simulink model "BLSMC"  (R2025b)
settings: Solver=ode3  StartTime=0.0  StopTime=1.5  FixedStep=1e-5  RelTol=1e-3  EnableMultiTasking=on
values from neighbouring files (symbols this model uses):
  beta = 2e3    (= 2000)    [plotting.m]    (also in robusnost_grafici.m)
  C = 470*10^-6    (= 0.00047)    [plotting.m]    (also in robusnost_grafici.m)
  k0 = 2*200    (= 400)    [plotting.m]    (also in robusnost_grafici.m)
  k1 = 1    [plotting.m]    (also in robusnost_grafici.m)
  ki = 200^2    (= 40000)    [plotting.m]    (also in robusnost_grafici.m)
  L = 15.91*10^-3    (= 0.01591)    [plotting.m]    (also in robusnost_grafici.m = 0.012728)
  poremecaj = 0.8    [plotting.m]    (also in robusnost_grafici.m)
  R = 52    [plotting.m]    (also in robusnost_grafici.m)
  sel = 3    [plotting.m]    (also in robusnost_grafici.m)
  sig2 = (0.02*x2e)^2    (= 0.2025)    [plotting.m]    (also in robusnost_grafici.m = 0)
  wp = 150    [plotting.m]    (also in robusnost_grafici.m)
  x2e = Vc    (= -22.5)    [plotting.m]    (also in robusnost_grafici.m)
settings Model: Creator=Stevica  LastModifiedBy=User
settings SolverCC: AlgebraicLoopSolver=TrustRegion
settings DataIOCC: LimitDataPoints=on  SaveFormat=Array
settings OptimizationCC: LifeSpan=inf
settings DebuggingCC: UnderspecifiedInitializationDetection=Classic  MergeDetectMultiDrivingBlocksExec=none  SolverPrmCheckMsg=warning  UnconnectedInputMsg=warning  UnconnectedOutputMsg=warning  UnconnectedLineMsg=warning  SFUnexpectedBacktrackingDiag=warning  SFNoUnconditionalDefaultTransitionDiag=warning  SFExecutionAtInitializationDiag=none  ArithmeticOperatorsInVariantConditions=warning
settings HardwareCC: ProdBitPerPointer=32.0  ProdBitPerSizeT=32.0  ProdBitPerPtrDiffT=32.0  ProdLargestAtomicFloat=None  ProdIntDivRoundTo=Undefined  ProdEndianess=Unspecified  ProdWordSize=32.0  ProdHWDeviceType=32-bit Generic
settings ModelReferenceCC: PropagateSignalLabelsOutOfModel=off
settings SFSimCC: SimUseLocalCustomCode=off  CustomCodeUndefinedFunction=UseInterfaceOnly
settings RTWCC: RTWUseLocalCustomCode=off  GPUComputeCapability=3.5
settings CodeAppCC: StateflowObjectComments=on
settings GRTTargetCC: TargetLangStandard=C89/C90 (ANSI)
settings ConfigComp: CovMetricSettings=dw  CovSaveCumulativeToWorkspaceVar=on  CovSaveSingleToWorkspaceVar=on  CovExternalEMLEnable=off

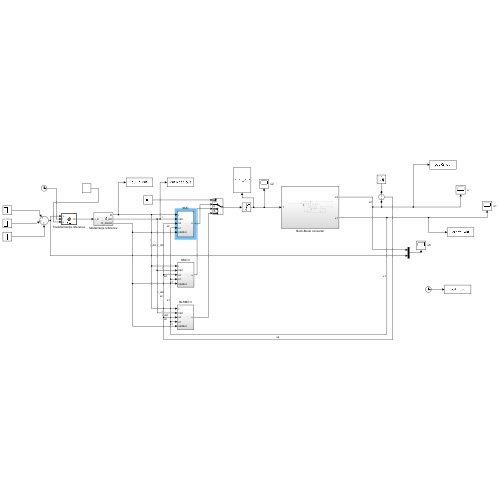
[thumbnail: Simulink's stored preview of the top-level diagram]
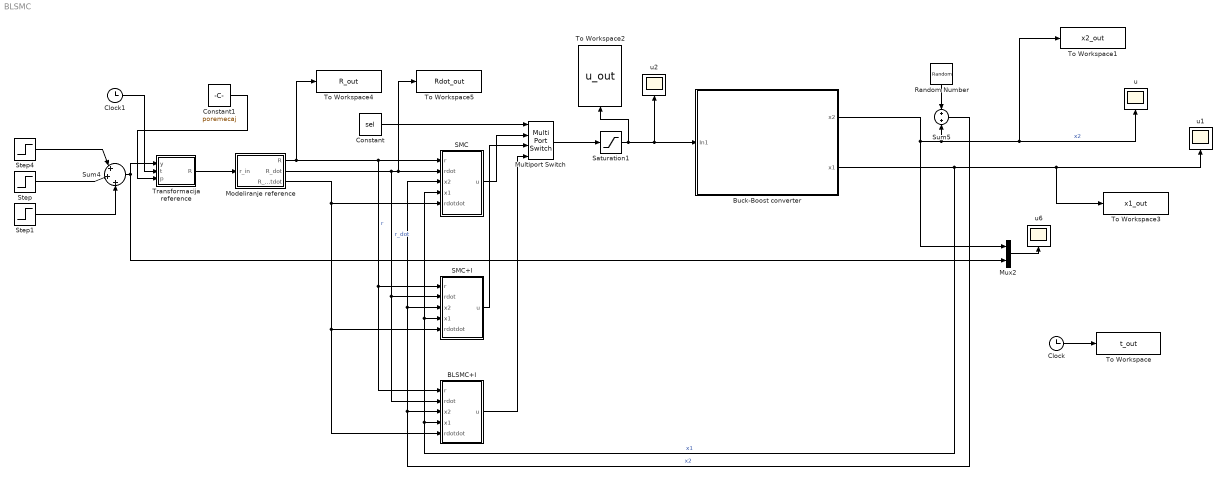
== system BLSMC ==
  BLSMC+I : Subsystem
      settings: PortSchema="{\"entries\":[{\"content\":{\"sides\":[{\"content\":{\"connectorIds\":[\"Out1\"]},\"type\":\"ConnectorPlacement.EquallySpacedRectSide\",\"uuid\":\"fc4d1246-7468-4525-a5ed-aeaa813f79b9\"},{\"content\":{\"connectorIds\":[\"In1\",\"In2\",\"In3\",\"In4\",\"In5\"],\"side\":\"RIGHT\"},\"type\":\"ConnectorPlacement.EquallySpacedRectSide\",\"uuid\":\"043d6a8f-e326-4119-9507-3ed5a55de0f4\"},{\"content\":{\"side\":\"TOP\"},\"type\":\"ConnectorPlacement.EquallySpacedRectSide\",\"uuid\":\"52d26304-56e6-4b52-8faf-a8e357024c95\"}]},\"type\":\"ConnectorPlacement.EquallySpacedConnector\",\"uuid\":\"d1c4fd68-439c-47cf-b9bf-33c74b646101\"}],\"packageUris\":[\"http://schema.mathworks.com/mf0/Connector/R2020b\"],\"version\":\"1.0\"}"
  Buck-Boost converter : Subsystem
  Clock : Clock
  Clock1 : Clock
  Constant : Constant  Value=sel
  Constant1 : Constant  Value=poremecaj
  Modeliranje reference : Subsystem
  Multiport Switch : MultiPortSwitch  SaturateOnIntegerOverflow=off  InputSameDT=off
  Mux2 : Mux  Inputs=2
  Random Number : RandomNumber  Variance=sig2  SampleTime=1e-5
  SMC : Subsystem
      settings: PortSchema="{\"entries\":[{\"content\":{\"sides\":[{\"content\":{\"connectorIds\":[\"Out1\"]},\"type\":\"ConnectorPlacement.EquallySpacedRectSide\",\"uuid\":\"fc4d1246-7468-4525-a5ed-aeaa813f79b9\"},{\"content\":{\"connectorIds\":[\"In1\",\"In2\",\"In3\",\"In4\",\"In5\"],\"side\":\"RIGHT\"},\"type\":\"ConnectorPlacement.EquallySpacedRectSide\",\"uuid\":\"043d6a8f-e326-4119-9507-3ed5a55de0f4\"},{\"content\":{\"side\":\"TOP\"},\"type\":\"ConnectorPlacement.EquallySpacedRectSide\",\"uuid\":\"52d26304-56e6-4b52-8faf-a8e357024c95\"}]},\"type\":\"ConnectorPlacement.EquallySpacedConnector\",\"uuid\":\"d1c4fd68-439c-47cf-b9bf-33c74b646101\"}],\"packageUris\":[\"http://schema.mathworks.com/mf0/Connector/R2020b\"],\"version\":\"1.0\"}"
  SMC+I : Subsystem
      settings: PortSchema="{\"entries\":[{\"content\":{\"sides\":[{\"content\":{\"connectorIds\":[\"Out1\"]},\"type\":\"ConnectorPlacement.EquallySpacedRectSide\",\"uuid\":\"fc4d1246-7468-4525-a5ed-aeaa813f79b9\"},{\"content\":{\"connectorIds\":[\"In1\",\"In2\",\"In3\",\"In4\",\"In5\"],\"side\":\"RIGHT\"},\"type\":\"ConnectorPlacement.EquallySpacedRectSide\",\"uuid\":\"043d6a8f-e326-4119-9507-3ed5a55de0f4\"},{\"content\":{\"side\":\"TOP\"},\"type\":\"ConnectorPlacement.EquallySpacedRectSide\",\"uuid\":\"52d26304-56e6-4b52-8faf-a8e357024c95\"}]},\"type\":\"ConnectorPlacement.EquallySpacedConnector\",\"uuid\":\"d1c4fd68-439c-47cf-b9bf-33c74b646101\"}],\"packageUris\":[\"http://schema.mathworks.com/mf0/Connector/R2020b\"],\"version\":\"1.0\"}"
  Saturation1 : Saturate  UpperLimit=1  LowerLimit=0
  Step : Step  Time=0.5  After=5  SampleTime=0
  Step1 : Step  After=-5  SampleTime=0
  Step4 : Step  Time=0  After=x2e  SampleTime=0
  Sum4 : Sum  Inputs=|+|+|+
  Sum5 : Sum
  To Workspace : ToWorkspace  VariableName=t_out  SampleTime=-1
  To Workspace1 : ToWorkspace  VariableName=x2_out  SampleTime=-1
  To Workspace2 : ToWorkspace  VariableName=u_out  SampleTime=-1
  To Workspace3 : ToWorkspace  VariableName=x1_out  SampleTime=-1
  To Workspace4 : ToWorkspace  VariableName=R_out  SampleTime=-1
  To Workspace5 : ToWorkspace  VariableName=Rdot_out  SampleTime=-1
  Transformacija reference : MATLAB Function  TreatAsAtomicUnit=on
  u{,1..2,6} (4 alike) : Scope
      u settings: ActiveDisplayYMinimum=-24.287940428418956  ActiveDisplayYMaximum=-16.345568269350679
      u1 settings: ActiveDisplayYMinimum=-0.56796240385681784  ActiveDisplayYMaximum=46.459814294123959
      u2 settings: ActiveDisplayYMinimum=0.31863871310778108  ActiveDisplayYMaximum=0.92761461889170183  DataLoggingVariableName=ScopeData3
      u6 settings: ActiveDisplayYMinimum=-24.906803320525466  ActiveDisplayYMaximum=-19.322890473907805  DataLoggingVariableName=ScopeData8
  wires:
  Buck-Boost converter/2(x1) -> To Workspace3/1, u1/1, BLSMC+I/4(x1), SMC/4(x1), SMC+I/4(x1)  "x1"
  Saturation1/1 -> Buck-Boost converter/1(In1), u2/1, To Workspace2/1
  Sum4/1 -> Mux2/2, Transformacija reference/1(y)
  Step/1 -> Sum4/2
  Step1/1 -> Sum4/3
  Sum5/1 -> BLSMC+I/3(x2), SMC/3(x2), SMC+I/3(x2)  "x2"
  Mux2/1 -> u6/1
  Step4/1 -> Sum4/1
  SMC/1(u) -> Multiport Switch/2
  Multiport Switch/1 -> Saturation1/1
  Modeliranje reference/1(R) -> To Workspace4/1, BLSMC+I/1(r), SMC+I/1(r), SMC/1(r)  "r"
  Modeliranje reference/2(R_dot) -> To Workspace5/1, SMC/2(rdot), BLSMC+I/2(rdot), SMC+I/2(rdot)  "r_dot"
  SMC+I/1(u) -> Multiport Switch/3
  BLSMC+I/1(u) -> Multiport Switch/4
  Constant/1 -> Multiport Switch/1
  Modeliranje reference/3(R_dotdot) -> SMC+I/5(rdotdot), BLSMC+I/5(rdotdot), SMC/5(rdotdot)
  Random Number/1 -> Sum5/1
  Buck-Boost converter/1(x2) -> Mux2/1, To Workspace1/1, u/1, Sum5/2  "x2"
  Clock/1 -> To Workspace/1
  Transformacija reference/1(R) -> Modeliranje reference/1(r_in)
  Clock1/1 -> Transformacija reference/2(t)
  Constant1/1 -> Transformacija reference/3(p)

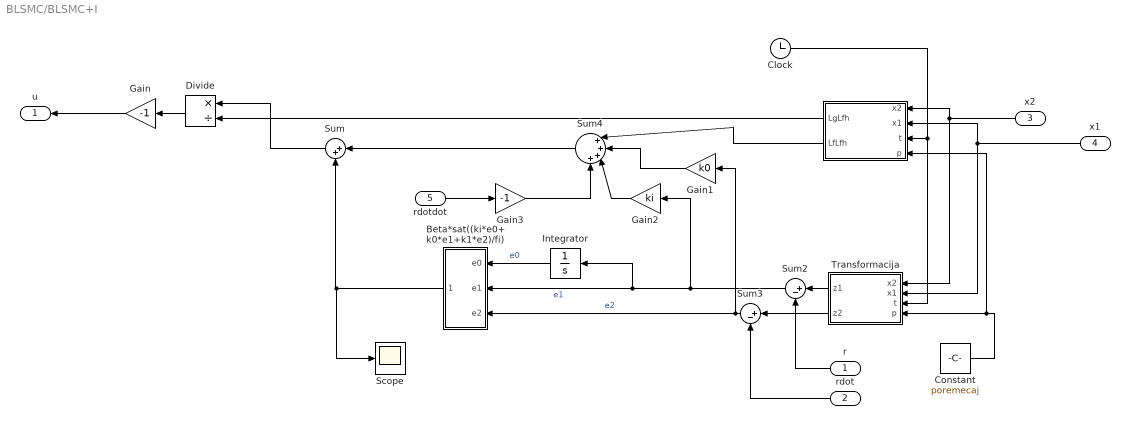
== system BLSMC/BLSMC+I ==
  r : Inport
  rdot : Inport  Port=2
  x2 : Inport  Port=3
  x1 : Inport  Port=4
  rdotdot : Inport  Port=5
  " " : MATLAB Function  TreatAsAtomicUnit=on
  Beta*sat((ki*e0+ k0*e1+k1*e2)/fi) : Subsystem
  Clock : Clock
  Constant : Constant  Value=poremecaj
  Divide : Product  Inputs=*/
  Gain : Gain  Gain=-1
  Gain1 : Gain  Gain=k0
  Gain2 : Gain  Gain=ki
  Gain3 : Gain  Gain=-1
  Integrator : Integrator
  Scope : Scope
      settings: ActiveDisplayYMinimum=-2170.4046249704252  ActiveDisplayYMaximum=-1714.2392861068972  DataLoggingVariableName=ScopeData4
  Sum : Sum  Inputs=|++
  Sum2 : Sum  Inputs=|+-
  Sum3 : Sum  Inputs=|+-
  Sum4 : Sum  Inputs=|++++
  Transformacija : MATLAB Function  TreatAsAtomicUnit=on
  u : Outport
  wires:
  Transformacija/1(z1) -> Sum2/1
  x2/1 -> Transformacija/1(x2), " "/1(x2)
  x1/1 -> Transformacija/2(x1), " "/2(x1)
  Transformacija/2(z2) -> Sum3/1
  Sum3/1 -> Gain1/1, Beta*sat((ki*e0+ k0*e1+k1*e2)/fi)/3(e2)  "e2"
  r/1 -> Sum2/2
  rdot/1 -> Sum3/2
  " "/2(LfLfh) -> Sum4/1
  Gain1/1 -> Sum4/2
  Sum4/1 -> Sum/1
  Sum2/1 -> Gain2/1, Integrator/1, Beta*sat((ki*e0+ k0*e1+k1*e2)/fi)/2(e1)  "e1"
  Beta*sat((ki*e0+ k0*e1+k1*e2)/fi)/1(Out1) -> Scope/1, Sum/2
  Sum/1 -> Divide/1
  " "/1(LgLfh) -> Divide/2
  Divide/1 -> Gain/1
  Gain/1 -> u/1
  Integrator/1 -> Beta*sat((ki*e0+ k0*e1+k1*e2)/fi)/1(e0)  "e0"
  Gain2/1 -> Sum4/3
  rdotdot/1 -> Gain3/1
  Gain3/1 -> Sum4/4
  Clock/1 -> Transformacija/3(t), " "/3(t)
  Constant/1 -> " "/4(p), Transformacija/4(p)

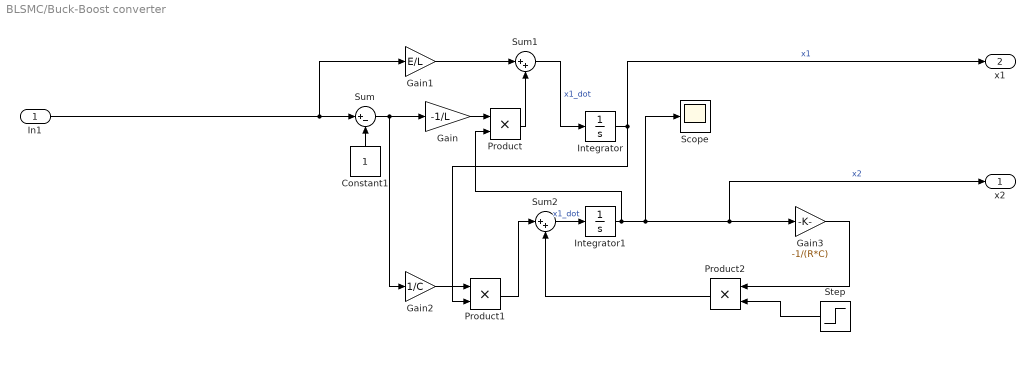
== system BLSMC/Buck-Boost converter ==
  In1 : Inport
  Constant1 : Constant
  Gain : Gain  Gain=-1/L
  Gain1 : Gain  Gain=E/L
  Gain2 : Gain  Gain=1/C
  Gain3 : Gain  Gain=-1/(R*C)
  Integrator : Integrator
  Integrator1 : Integrator
  Product : Product
  Product1 : Product
  Product2 : Product
  Scope : Scope
      settings: ActiveDisplayYMinimum=-25.046281735862888  ActiveDisplayYMaximum=-15.447926718255747  DataLoggingVariableName=ScopeData8
  Step : Step  Time=1.3  Before=1  After=1/poremecaj  SampleTime=0
  Sum : Sum  Inputs=|+-
  Sum1 : Sum  Inputs=|++
  Sum2 : Sum  Inputs=|++
  x2 : Outport
  x1 : Outport  Port=2
  wires:
  Gain/1 -> Product/1
  In1/1 -> Gain1/1, Sum/1
  Sum1/1 -> Integrator/1  "x1_dot"
  Gain1/1 -> Sum1/1
  Sum/1 -> Gain2/1, Gain/1
  Constant1/1 -> Sum/2
  Gain2/1 -> Product1/1
  Product/1 -> Sum1/2
  Integrator1/1 -> x2/1, Gain3/1, Scope/1, Product/2  "x2"
  Product1/1 -> Sum2/1
  Integrator/1 -> x1/1, Product1/2  "x1"
  Sum2/1 -> Integrator1/1  "x1_dot"
  Gain3/1 -> Product2/1
  Product2/1 -> Sum2/2
  Step/1 -> Product2/2

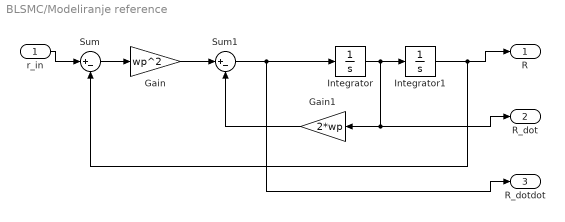
== system BLSMC/Modeliranje reference ==
  r_in : Inport
  Gain : Gain  Gain=wp^2
  Gain1 : Gain  Gain=2*wp
  Integrator : Integrator
  Integrator1 : Integrator
  Sum : Sum  Inputs=|+-
  Sum1 : Sum  Inputs=|+-
  R : Outport
  R_dot : Outport  Port=2
  R_dotdot : Outport  Port=3
  wires:
  r_in/1 -> Sum/1
  Sum/1 -> Gain/1
  Gain/1 -> Sum1/1
  Integrator/1 -> R_dot/1, Gain1/1, Integrator1/1
  Integrator1/1 -> Sum/2, R/1
  Gain1/1 -> Sum1/2
  Sum1/1 -> R_dotdot/1, Integrator/1

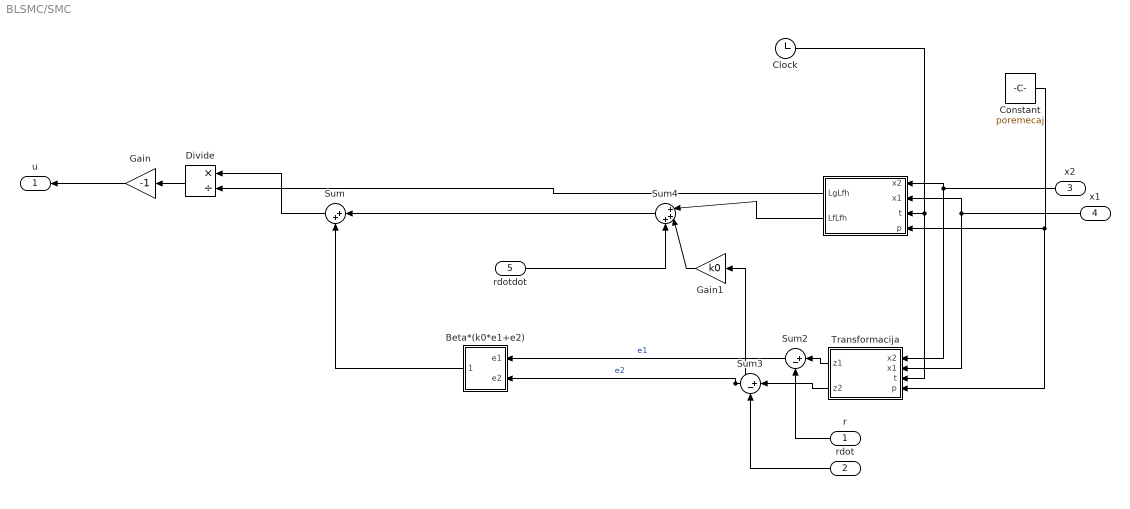
== system BLSMC/SMC ==
  r : Inport
  rdot : Inport  Port=2
  x2 : Inport  Port=3
  x1 : Inport  Port=4
  rdotdot : Inport  Port=5
  " " : MATLAB Function  TreatAsAtomicUnit=on
  Beta*(k0*e1+e2) : Subsystem
  Clock : Clock
  Constant : Constant  Value=poremecaj
  Divide : Product  Inputs=*/
  Gain : Gain  Gain=-1
  Gain1 : Gain  Gain=k0
  Sum : Sum  Inputs=|++
  Sum2 : Sum  Inputs=|+-
  Sum3 : Sum  Inputs=|+-
  Sum4 : Sum  Inputs=|+++
  Transformacija : MATLAB Function  TreatAsAtomicUnit=on
  u : Outport
  wires:
  Transformacija/1(z1) -> Sum2/1
  x2/1 -> Transformacija/1(x2), " "/1(x2)
  x1/1 -> " "/2(x1), Transformacija/2(x1)
  Transformacija/2(z2) -> Sum3/1
  Sum3/1 -> Beta*(k0*e1+e2)/2(e2), Gain1/1  "e2"
  r/1 -> Sum2/2
  rdot/1 -> Sum3/2
  " "/2(LfLfh) -> Sum4/1
  Gain1/1 -> Sum4/2
  Sum4/1 -> Sum/1
  Sum2/1 -> Beta*(k0*e1+e2)/1(e1)  "e1"
  Beta*(k0*e1+e2)/1(Out1) -> Sum/2
  Sum/1 -> Divide/1
  " "/1(LgLfh) -> Divide/2
  Divide/1 -> Gain/1
  Gain/1 -> u/1
  rdotdot/1 -> Sum4/3
  Clock/1 -> Transformacija/3(t), " "/3(t)
  Constant/1 -> Transformacija/4(p), " "/4(p)

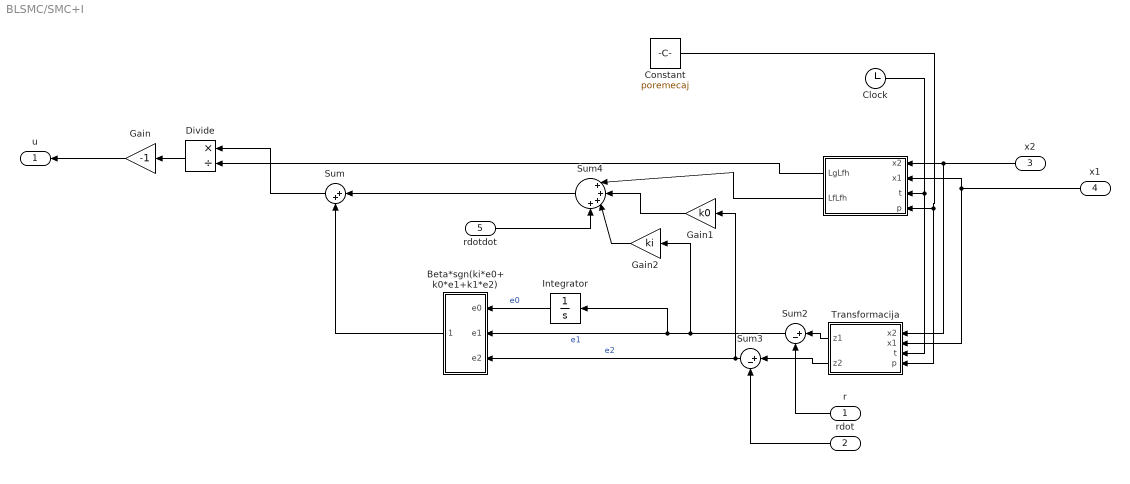
== system BLSMC/SMC+I ==
  r : Inport
  rdot : Inport  Port=2
  x2 : Inport  Port=3
  x1 : Inport  Port=4
  rdotdot : Inport  Port=5
  " " : MATLAB Function  TreatAsAtomicUnit=on
  Beta*sgn(ki*e0+ k0*e1+k1*e2) : Subsystem
  Clock : Clock
  Constant : Constant  Value=poremecaj
  Divide : Product  Inputs=*/
  Gain : Gain  Gain=-1
  Gain1 : Gain  Gain=k0
  Gain2 : Gain  Gain=ki
  Integrator : Integrator
  Sum : Sum  Inputs=|++
  Sum2 : Sum  Inputs=|+-
  Sum3 : Sum  Inputs=|+-
  Sum4 : Sum  Inputs=|++++
  Transformacija : MATLAB Function  TreatAsAtomicUnit=on
  u : Outport
  wires:
  Transformacija/1(z1) -> Sum2/1
  x2/1 -> Transformacija/1(x2), " "/1(x2)
  x1/1 -> " "/2(x1), Transformacija/2(x1)
  Transformacija/2(z2) -> Sum3/1
  Sum3/1 -> Gain1/1, Beta*sgn(ki*e0+ k0*e1+k1*e2)/3(e2)  "e2"
  r/1 -> Sum2/2
  rdot/1 -> Sum3/2
  " "/2(LfLfh) -> Sum4/1
  Gain1/1 -> Sum4/2
  Sum4/1 -> Sum/1
  Sum2/1 -> Gain2/1, Integrator/1, Beta*sgn(ki*e0+ k0*e1+k1*e2)/2(e1)  "e1"
  Beta*sgn(ki*e0+ k0*e1+k1*e2)/1(Out1) -> Sum/2
  Sum/1 -> Divide/1
  " "/1(LgLfh) -> Divide/2
  Divide/1 -> Gain/1
  Gain/1 -> u/1
  Integrator/1 -> Beta*sgn(ki*e0+ k0*e1+k1*e2)/1(e0)  "e0"
  Gain2/1 -> Sum4/3
  rdotdot/1 -> Sum4/4
  Clock/1 -> Transformacija/3(t), " "/3(t)
  Constant/1 -> Transformacija/4(p), " "/4(p)

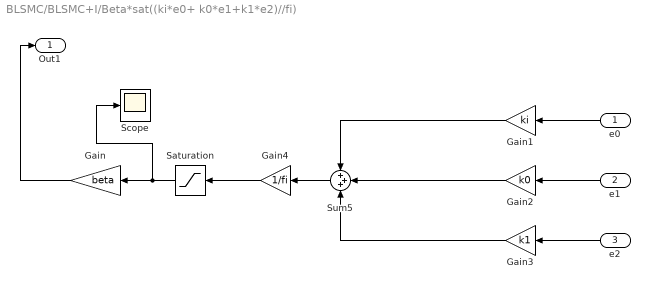
== system BLSMC/BLSMC+I/Beta*sat((ki*e0+ k0*e1+k1*e2)//fi) ==
  e0 : Inport
  e1 : Inport  Port=2
  e2 : Inport  Port=3
  Gain : Gain  Gain=beta
  Gain1 : Gain  Gain=ki
  Gain2 : Gain  Gain=k0
  Gain3 : Gain  Gain=k1
  Gain4 : Gain  Gain=1/fi
  Saturation : Saturate  UpperLimit=1  LowerLimit=-1
  Scope : Scope
      settings: ActiveDisplayYMinimum=-4.0472642179198353  ActiveDisplayYMaximum=4.3871527582806635  DataLoggingVariableName=ScopeData2
  Sum5 : Sum  Inputs=+++
  Out1 : Outport
  wires:
  Gain2/1 -> Sum5/2
  Sum5/1 -> Gain4/1
  Saturation/1 -> Scope/1, Gain/1
  e1/1 -> Gain2/1
  Gain/1 -> Out1/1
  e2/1 -> Gain3/1
  e0/1 -> Gain1/1
  Gain1/1 -> Sum5/1
  Gain3/1 -> Sum5/3
  Gain4/1 -> Saturation/1

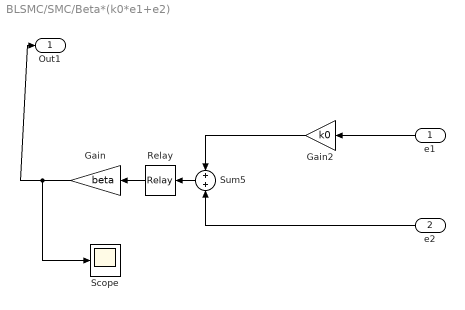
== system BLSMC/SMC/Beta*(k0*e1+e2) ==
  e1 : Inport
  e2 : Inport  Port=2
  Gain : Gain  Gain=beta
  Gain2 : Gain  Gain=k0
  Relay : Relay  OnSwitchValue=0  OffSwitchValue=0  OffOutputValue=-1
  Scope : Scope
      settings: ActiveDisplayYMinimum=-35.428031852523034  ActiveDisplayYMaximum=51.802721406020112  DataLoggingVariableName=ScopeData5
  Sum5 : Sum  Inputs=+|+
  Out1 : Outport
  wires:
  Gain2/1 -> Sum5/1
  Sum5/1 -> Relay/1
  Relay/1 -> Gain/1
  e1/1 -> Gain2/1
  Gain/1 -> Scope/1, Out1/1
  e2/1 -> Sum5/2

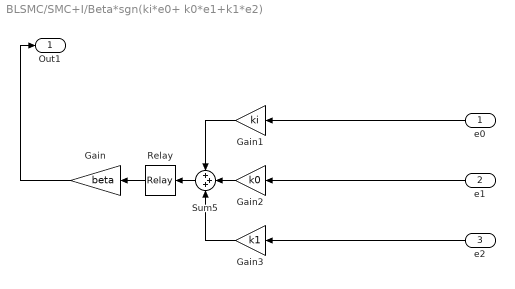
== system BLSMC/SMC+I/Beta*sgn(ki*e0+ k0*e1+k1*e2) ==
  e0 : Inport
  e1 : Inport  Port=2
  e2 : Inport  Port=3
  Gain : Gain  Gain=beta
  Gain1 : Gain  Gain=ki
  Gain2 : Gain  Gain=k0
  Gain3 : Gain  Gain=k1
  Relay : Relay  OnSwitchValue=0  OffSwitchValue=0  OffOutputValue=-1
  Sum5 : Sum  Inputs=+++
  Out1 : Outport
  wires:
  Gain2/1 -> Sum5/2
  Sum5/1 -> Relay/1
  Relay/1 -> Gain/1
  e1/1 -> Gain2/1
  Gain/1 -> Out1/1
  e2/1 -> Gain3/1
  e0/1 -> Gain1/1
  Gain1/1 -> Sum5/1
  Gain3/1 -> Sum5/3

== matlab function BLSMC/SMC/Transformacija ==
  data: x2 input; z1 output; x1 input; z2 output; t input; p input
function [z1, z2] = fcn(x2, x1, t, p)

L=15.91*10^-3;
C=470*10^-6;
if t < 1.3
    R = 52;
else
    R = 52*p;
end
E=12;

Vc=-22.5;
x2e=Vc;
x1e=1.2441;


z1 = C*x2^2 - 2*E*C*x2 + L*x1^2 + C*E^2 - (C*x2e^2 - 2*E*C*x2e + L*x1e^2 + C*E^2);
z2 = -2/R*x2^2 + 2*E*x1 + 2*E/R*x2;

== matlab function BLSMC/SMC/  ==
  data: x2 input; LgLfh output; x1 input; LfLfh output; t input; p input
function [LgLfh, LfLfh] = fcn(x2, x1, t, p)

L=15.91*10^-3;
C=470*10^-6;
if t < 1.3
    R = 52;
else
    R = 52*p;
end
E=12;

LgLfh = -4/(R*C)*x2*x1 + 2*E/(R*C)*x1 + 2*E^2/L - 2*E/L*x2;
LfLfh = 4/(R^2*C)*x2^2 - 2*E/(R^2*C)*x2 + 2*E/L*x2...
    - 2*E/(R*C)*x1 +4/(R*C)*x2*x1;

== matlab function BLSMC/Transformacija reference ==
  data: y input; R output; t input; p input
function  R= fcn(y, t, p)

% y=x1e stara referenca, tj. nominalna vrednost

L=15.91*10^-3;
C=470*10^-6;
if t < 1.3
    R = 52;
else
    R = 52*p;
end
E=12;

Vc=-22.5;
x2e=Vc;
x1e=1.2441;

gama = C*x2e^2 - 2*E*C*x2e + L*x1e^2;

R = C*y^2 - 2*E*C*y + L*(y*(y-E)/(R*E))^2 - gama;

== matlab function BLSMC/SMC+I/  ==
  data: x2 input; LgLfh output; x1 input; LfLfh output; t input; p input
function [LgLfh, LfLfh] = fcn(x2, x1, t, p)

L=15.91*10^-3;
C=470*10^-6;
if t < 1.3
    R = 52;
else
    R = 52*p;
end
E=12;

LgLfh = -4/(R*C)*x2*x1 + 2*E/(R*C)*x1 + 2*E^2/L - 2*E/L*x2;
LfLfh = 4/(R^2*C)*x2^2 - 2*E/(R^2*C)*x2 + 2*E/L*x2...
    - 2*E/(R*C)*x1 +4/(R*C)*x2*x1;

== matlab function BLSMC/SMC+I/Transformacija ==
  data: x2 input; z1 output; x1 input; z2 output; t input; p input
function [z1, z2] = fcn(x2, x1, t, p)

L=15.91*10^-3;
C=470*10^-6;
if t < 1.3
    R = 52;
else
    R = 52*p;
end
E=12;

Vc=-22.5;
x2e=Vc;
x1e=1.2441;


z1 = C*x2^2 - 2*E*C*x2 + L*x1^2 + C*E^2 - (C*x2e^2 - 2*E*C*x2e + L*x1e^2 + C*E^2);
z2 = -2/R*x2^2 + 2*E*x1 + 2*E/R*x2;

== matlab function BLSMC/BLSMC+I/  ==
  data: x2 input; LgLfh output; x1 input; LfLfh output; t input; p input
function [LgLfh, LfLfh] = fcn(x2, x1, t, p)

L=15.91*10^-3;
C=470*10^-6;
if t < 1.3
    R = 52;
else
    R = 52*p;
end

E=12;

LgLfh = -4/(R*C)*x2*x1 + 2*E/(R*C)*x1 + 2*E^2/L - 2*E/L*x2;
LfLfh = 4/(R^2*C)*x2^2 - 2*E/(R^2*C)*x2 + 2*E/L*x2...
    - 2*E/(R*C)*x1 +4/(R*C)*x2*x1;

== matlab function BLSMC/BLSMC+I/Transformacija ==
  data: x2 input; x1 input; z1 output; z2 output; t input; p input
function [z1, z2] = fcn(x2, x1, t, p)

L=15.91*10^-3;
C=470*10^-6;
if t < 1.3
    R = 52;
else
    R = 52*p;
end

E=12;

Vc=-22.5;
x2e=Vc;
x1e=1.2441;


z1 = C*x2^2 - 2*E*C*x2 + L*x1^2 + C*E^2 - (C*x2e^2 - 2*E*C*x2e + L*x1e^2 + C*E^2);
z2 = -2/R*x2^2 + 2*E*x1 + 2*E/R*x2;
